simulink model "EKFSCARA"  (Simulink 8.1)
settings: Solver=ode3  StartTime=0.0  StopTime=100  FixedStep=.1  RelTol=1e-3
libraries: roblocks x1
settings Model: Creator=mahyar  LastModifiedBy=mahyar
settings DataIOCC: SignalLoggingSaveFormat=Dataset
settings OptimizationCC: ExpressionDepthLimit=128
settings DebuggingCC: FcnCallInpInsideContextMsg=EnableAllAsError
settings GRTTargetCC: CombineOutputUpdateFcns=on  GRTInterface=off

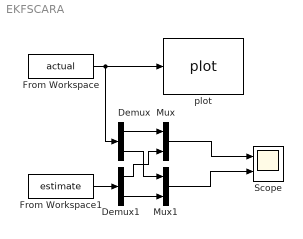
== system EKFSCARA ==
  Demux : Demux  Outputs=2
  Demux1 : Demux  Outputs=2
  From Workspace : FromWorkspace  VariableName=actual  SampleTime=0
  From Workspace1 : FromWorkspace  VariableName=estimate  SampleTime=0
  Mux : Mux  Inputs=2
  Mux1 : Mux  Inputs=2
  Scope : Scope  NumInputPorts=2
      settings: TimeRange=100  YMin=-0.9~-0.9  YMax=1~1
  plot : roblocks/plot  robot=r
  wires:
  From Workspace/1 -> Demux/1, plot/1
  Mux/1 -> Scope/1
  Mux1/1 -> Scope/2
  From Workspace1/1 -> Demux1/1
  Demux/1 -> Mux/1
  Demux1/2 -> Mux1/2
  Demux/2 -> Mux1/1
  Demux1/1 -> Mux/2
